simulink model "CDA"  (R2020a)
settings: Solver=VariableStepAuto  StartTime=0.0  StopTime=300  RelTol=1e-9
values from neighbouring files (symbols this model uses):
  bp = 0.05    [simulacion.m]
  kp = 3.0    (= 3)    [simulacion.m]
  kp_poc = 0.4    [simulacion.m]
  P_i_u1 = SP1    (= 180)    [simulacion.m]
  P_i_u2 = P2(1)    [simulacion.m]
  P_i_u3 = P3(1)    [simulacion.m]
  q_i_u1 = condiciones.q_i    [simulacion.m]
  q_i_u2 = condiciones.q_i    [simulacion.m]
  q_i_u3 = condiciones.q_i    [simulacion.m]
  qt_i = q_i_u1 + q_i_u2 + q_i_u3    [simulacion.m]
  SP1 = 180    [simulacion.m]
  SP2 = 180    [simulacion.m]
  SP3 = 180    [simulacion.m]
  t3 = 0.01    [simulacion.m]
  td = 0    [simulacion.m]
  tn_poc = 5    [simulacion.m]
  tx = 0.8    [simulacion.m]
  y_i_u1 = condiciones.y_i    [simulacion.m]
  y_i_u2 = condiciones.y_i    [simulacion.m]
  y_i_u3 = condiciones.y_i    [simulacion.m]
libraries: simulink x6, simulink_extras x6
settings Model: Creator=Lenovo  LastModifiedBy=Lenovo
settings SolverCC: AlgebraicLoopSolver=LineSearch

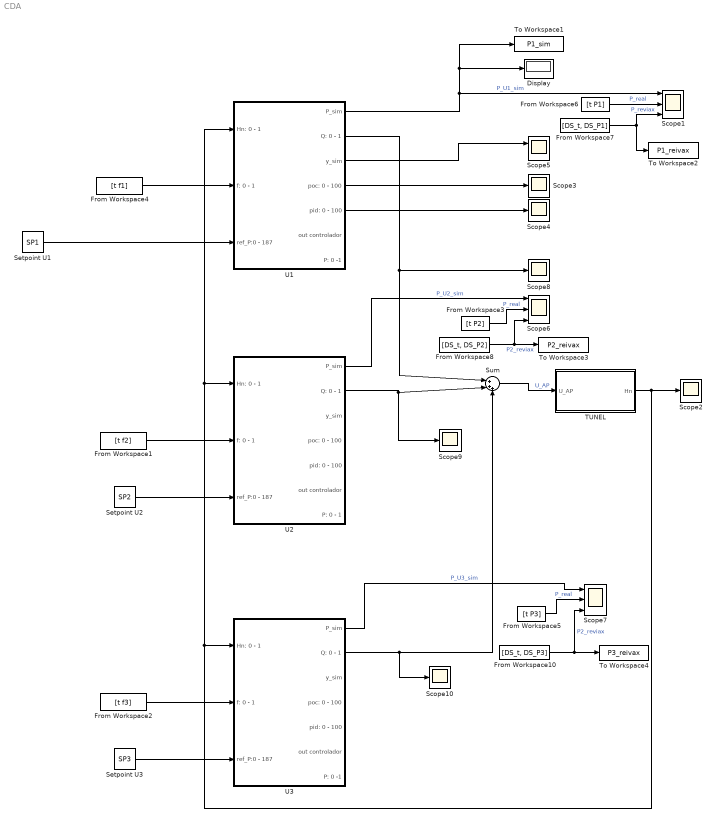
== system CDA ==
  Display : Display
  From Workspace1 : FromWorkspace  VariableName=[t f2]
  From Workspace10 : FromWorkspace  VariableName=[DS_t, DS_P3]
  From Workspace2 : FromWorkspace  VariableName=[t f3]
  From Workspace3 : FromWorkspace  VariableName=[t P2]
  From Workspace4 : FromWorkspace  VariableName=[t f1]
  From Workspace5 : FromWorkspace  VariableName=[t P3]
  From Workspace6 : FromWorkspace  VariableName=[t P1]
  From Workspace7 : FromWorkspace  VariableName=[DS_t, DS_P1]
  From Workspace8 : FromWorkspace  VariableName=[DS_t, DS_P2]
  Scope1 : Scope  NumInputPorts=3
  Scope{2..4,8..10} (6 alike) : Scope
  Scope5 : Scope  NumInputPorts=2
  Scope6 : Scope  NumInputPorts=3
  Scope7 : Scope  NumInputPorts=3
  Setpoint U1 : Constant  Value=SP1
  Setpoint U2 : Constant  Value=SP2
  Setpoint U3 : Constant  Value=SP3
  Sum : Sum  Inputs=|+++
  TUNEL : Subsystem
  To Workspace1 : ToWorkspace  VariableName=P1_sim  SaveFormat=Timeseries  SampleTime=1
  To Workspace2 : ToWorkspace  VariableName=P1_reivax  SaveFormat=Timeseries  SampleTime=1
  To Workspace3 : ToWorkspace  VariableName=P2_reivax  SaveFormat=Timeseries  SampleTime=1
  To Workspace4 : ToWorkspace  VariableName=P3_reivax  SaveFormat=Timeseries  SampleTime=1
  U1 : Subsystem
  U2 : Subsystem
  U3 : Subsystem
  wires:
  From Workspace6/1 -> Scope1/2  "P_real"
  U1/1(P_sim) -> To Workspace1/1, Display/1, Scope1/1  "P_U1_sim"
  From Workspace4/1 -> U1/2(f: 0 - 1)
  Setpoint U1/1 -> U1/3(ref_P:0 - 187)
  U1/3(y_sim) -> Scope5/1
  U1/4(poc: 0 - 100) -> Scope3/1
  U1/5(pid: 0 - 100) -> Scope4/1
  U1/2(Q: 0 - 1) -> Sum/1, Scope8/1
  U2/2(Q: 0 - 1) -> Scope9/1, Sum/2
  U3/2(Q: 0 - 1) -> Sum/3, Scope10/1
  TUNEL/1(Hn) -> Scope2/1, U1/1(Hn: 0 - 1), U2/1(Hn: 0 - 1), U3/1(Hn: 0 - 1)
  Sum/1 -> TUNEL/1(U_AP)  "U_AP"
  Setpoint U2/1 -> U2/3(ref_P:0 - 187)
  Setpoint U3/1 -> U3/3(ref_P:0 - 187)
  U2/1(P_sim) -> Scope6/1  "P_U2_sim"
  From Workspace3/1 -> Scope6/2  "P_real"
  From Workspace5/1 -> Scope7/2  "P_real"
  U3/1(P_sim) -> Scope7/1  "P_U3_sim"
  From Workspace7/1 -> Scope1/3, To Workspace2/1  "P_reviax"
  From Workspace1/1 -> U2/2(f: 0 - 1)
  From Workspace2/1 -> U3/2(f: 0 - 1)
  From Workspace8/1 -> To Workspace3/1, Scope6/3  "P2_reviax"
  From Workspace10/1 -> Scope7/3, To Workspace4/1  "P2_reviax"

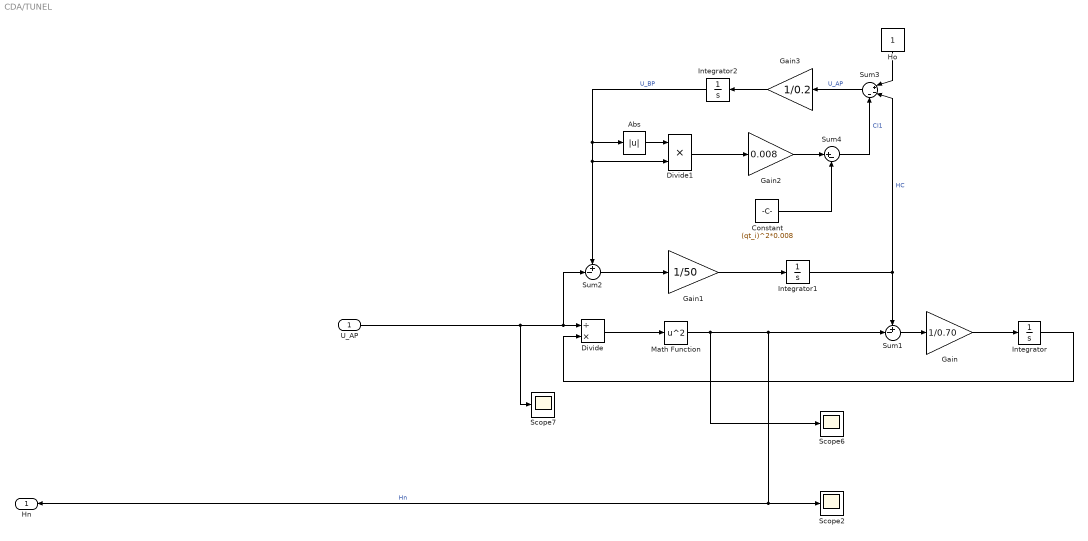
== system CDA/TUNEL ==
  U_AP : Inport
  Abs : Abs
  Constant : Constant  Value=(qt_i)^2*0.008
  Divide : Product  Inputs=/*
  Divide1 : Product  Inputs=**
  Gain : Gain  Gain=1/0.70
  Gain1 : Gain  Gain=1/50
  Gain2 : Gain  Gain=0.008
  Gain3 : Gain  Gain=1/0.2
  Ho : Constant
  Integrator : Integrator  InitialCondition=qt_i
  Integrator1 : Integrator  InitialCondition=1
  Integrator2 : Integrator  InitialCondition=qt_i
  Math Function : Math  Operator=square  SaturateOnIntegerOverflow=on
  Scope2 : Scope
  Scope6 : Scope
  Scope7 : Scope
  Sum1 : Sum  Inputs=+-|
  Sum2 : Sum  Inputs=+-|
  Sum3 : Sum  Inputs=|+--
  Sum4 : Sum  Inputs=|+-
  Hn : Outport
  wires:
  Math Function/1 -> Scope6/1, Hn/1, Scope2/1, Sum1/2  "Hn"
  Gain1/1 -> Integrator1/1
  Integrator2/1 -> Abs/1, Divide1/2, Sum2/1  "U_BP"
  Ho/1 -> Sum3/1
  Integrator/1 -> Divide/2
  Gain/1 -> Integrator/1
  Divide/1 -> Math Function/1
  Sum4/1 -> Sum3/3  "CI1"
  U_AP/1 -> Scope7/1, Sum2/2, Divide/1
  Gain2/1 -> Sum4/1
  Integrator1/1 -> Sum3/2, Sum1/1  "HC"
  Constant/1 -> Sum4/2
  Sum1/1 -> Gain/1
  Gain3/1 -> Integrator2/1
  Sum2/1 -> Gain1/1
  Divide1/1 -> Gain2/1
  Sum3/1 -> Gain3/1  "U_AP"
  Abs/1 -> Divide1/1

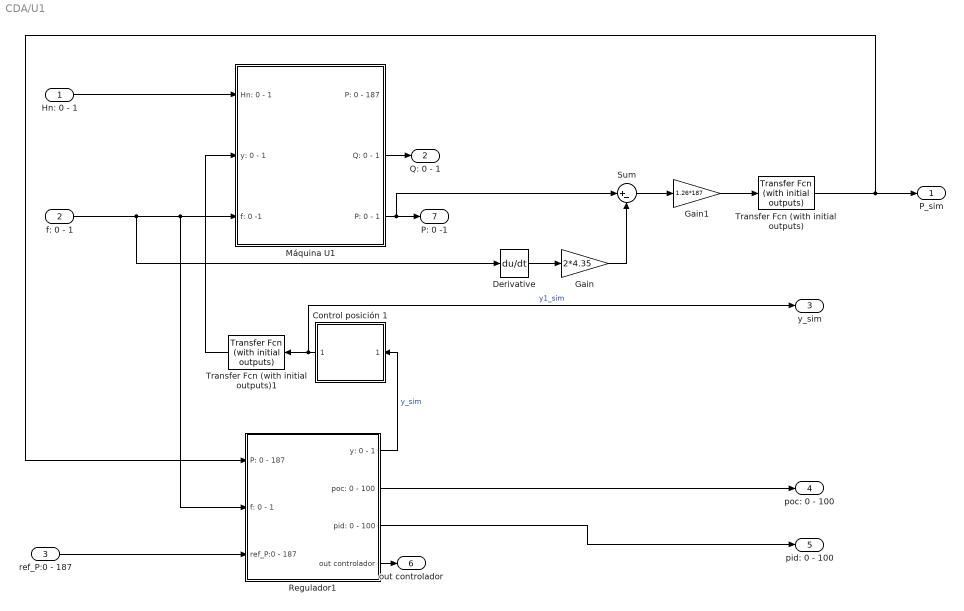
== system CDA/U1 ==
  Hn: 0 - 1 : Inport
  f: 0 - 1 : Inport  Port=2
  ref_P:0 - 187 : Inport  Port=3
  Control posición 1 : Subsystem
  Derivative : Derivative
  Gain : Gain  Gain=2*4.35
  Gain1 : Gain  Gain=1.26*187
  Máquina U1 : Subsystem
  Regulador1 : Subsystem
  Sum : Sum  Inputs=|+-
  Transfer Fcn (with initial outputs) : simulink_extras/Additional Linear/Transfer Fcn (with initial outputs)  N=[1]  D="[0.2  1]"  Y0=P_i_u1  U0=P_i_u1/(1.26*187)
  Transfer Fcn (with initial outputs)1 : simulink_extras/Additional Linear/Transfer Fcn (with initial outputs)  N=[1]  D=[1e-6 1]  Y0=y_i_u1  U0=y_i_u1
  P_sim : Outport
  Q: 0 - 1 : Outport  Port=2
  y_sim : Outport  Port=3
  poc: 0 - 100 : Outport  Port=4
  pid: 0 - 100 : Outport  Port=5
  out controlador : Outport  Port=6
  P: 0 -1 : Outport  Port=7
  wires:
  Control posición 1/1(yr: 0 - 1) -> Transfer Fcn (with initial outputs)1/1, y_sim/1  "y1_sim"
  Regulador1/1(y: 0 - 1) -> Control posición 1/1(yf: 0 - 1)  "y_sim"
  Máquina U1/2(Q: 0 - 1) -> Q: 0 - 1/1
  ref_P:0 - 187/1 -> Regulador1/3(ref_P:0 - 187)
  Hn: 0 - 1/1 -> Máquina U1/1(Hn: 0 - 1)
  f: 0 - 1/1 -> Derivative/1, Máquina U1/3(f: 0 -1), Regulador1/2(f: 0 - 1)
  Transfer Fcn (with initial outputs)1/1 -> Máquina U1/2(y: 0 - 1)
  Regulador1/3(pid: 0 - 100) -> pid: 0 - 100/1
  Regulador1/2(poc: 0 - 100) -> poc: 0 - 100/1
  Regulador1/4(out controlador) -> out controlador/1
  Máquina U1/3(P: 0 - 1) -> Sum/1, P: 0 -1/1
  Derivative/1 -> Gain/1
  Gain/1 -> Sum/2
  Sum/1 -> Gain1/1
  Gain1/1 -> Transfer Fcn (with initial outputs)/1
  Transfer Fcn (with initial outputs)/1 -> Regulador1/1(P: 0 - 187), P_sim/1

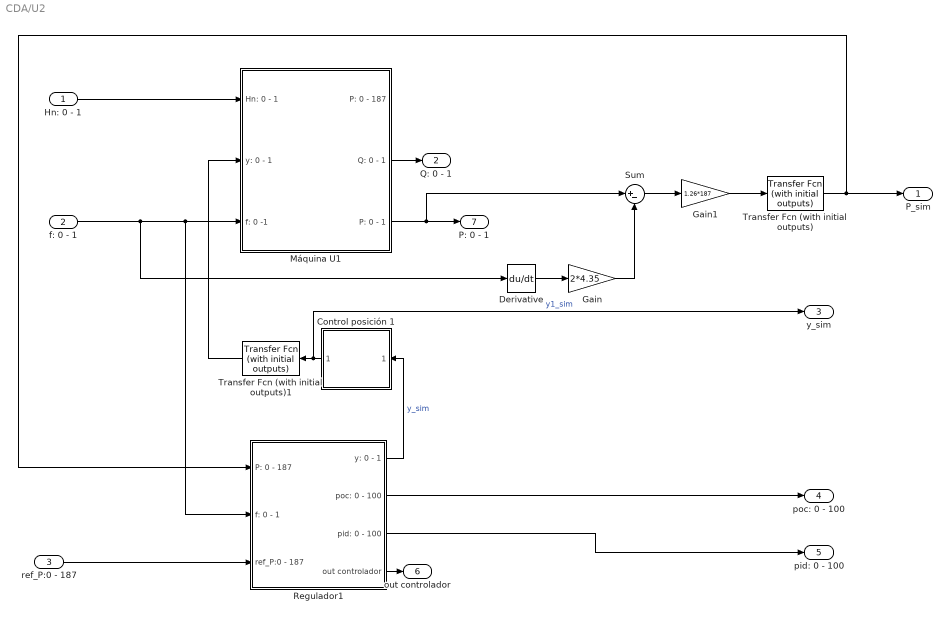
== system CDA/U2 ==
  Hn: 0 - 1 : Inport
  f: 0 - 1 : Inport  Port=2
  ref_P:0 - 187 : Inport  Port=3
  Control posición 1 : Subsystem
  Derivative : Derivative
  Gain : Gain  Gain=2*4.35
  Gain1 : Gain  Gain=1.26*187
  Máquina U1 : Subsystem
  Regulador1 : Subsystem
  Sum : Sum  Inputs=|+-
  Transfer Fcn (with initial outputs) : simulink_extras/Additional Linear/Transfer Fcn (with initial outputs)  N=[1]  D="[0.2  1]"  Y0=P_i_u2  U0=P_i_u2/(1.26*187)
  Transfer Fcn (with initial outputs)1 : simulink_extras/Additional Linear/Transfer Fcn (with initial outputs)  N=[1]  D=[1e-6 1]  Y0=y_i_u2  U0=y_i_u2
  P_sim : Outport
  Q: 0 - 1 : Outport  Port=2
  y_sim : Outport  Port=3
  poc: 0 - 100 : Outport  Port=4
  pid: 0 - 100 : Outport  Port=5
  out controlador : Outport  Port=6
  P: 0 - 1 : Outport  Port=7
  wires:
  Control posición 1/1(yr: 0 - 1) -> Transfer Fcn (with initial outputs)1/1, y_sim/1  "y1_sim"
  Regulador1/1(y: 0 - 1) -> Control posición 1/1(yf: 0 - 1)  "y_sim"
  Máquina U1/2(Q: 0 - 1) -> Q: 0 - 1/1
  ref_P:0 - 187/1 -> Regulador1/3(ref_P:0 - 187)
  Hn: 0 - 1/1 -> Máquina U1/1(Hn: 0 - 1)
  Transfer Fcn (with initial outputs)1/1 -> Máquina U1/2(y: 0 - 1)
  Regulador1/3(pid: 0 - 100) -> pid: 0 - 100/1
  Regulador1/2(poc: 0 - 100) -> poc: 0 - 100/1
  Regulador1/4(out controlador) -> out controlador/1
  Máquina U1/3(P: 0 - 1) -> Sum/1, P: 0 - 1/1
  Sum/1 -> Gain1/1
  Gain/1 -> Sum/2
  Derivative/1 -> Gain/1
  f: 0 - 1/1 -> Derivative/1, Máquina U1/3(f: 0 -1), Regulador1/2(f: 0 - 1)
  Gain1/1 -> Transfer Fcn (with initial outputs)/1
  Transfer Fcn (with initial outputs)/1 -> P_sim/1, Regulador1/1(P: 0 - 187)

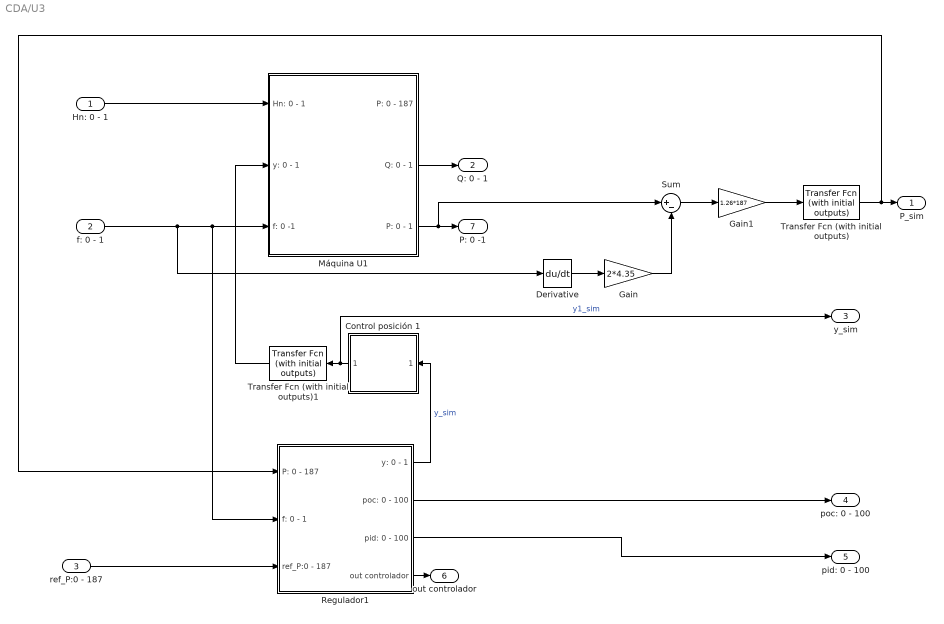
== system CDA/U3 ==
  Hn: 0 - 1 : Inport
  f: 0 - 1 : Inport  Port=2
  ref_P:0 - 187 : Inport  Port=3
  Control posición 1 : Subsystem
  Derivative : Derivative
  Gain : Gain  Gain=2*4.35
  Gain1 : Gain  Gain=1.26*187
  Máquina U1 : Subsystem
  Regulador1 : Subsystem
  Sum : Sum  Inputs=|+-
  Transfer Fcn (with initial outputs) : simulink_extras/Additional Linear/Transfer Fcn (with initial outputs)  N=[1]  D="[0.2  1]"  Y0=P_i_u3  U0=P_i_u3/(1.26*187)
  Transfer Fcn (with initial outputs)1 : simulink_extras/Additional Linear/Transfer Fcn (with initial outputs)  N=[1]  D=[1e-6 1]  Y0=y_i_u3  U0=y_i_u3
  P_sim : Outport
  Q: 0 - 1 : Outport  Port=2
  y_sim : Outport  Port=3
  poc: 0 - 100 : Outport  Port=4
  pid: 0 - 100 : Outport  Port=5
  out controlador : Outport  Port=6
  P: 0 -1 : Outport  Port=7
  wires:
  Control posición 1/1(yr: 0 - 1) -> Transfer Fcn (with initial outputs)1/1, y_sim/1  "y1_sim"
  Regulador1/1(y: 0 - 1) -> Control posición 1/1(yf: 0 - 1)  "y_sim"
  Máquina U1/2(Q: 0 - 1) -> Q: 0 - 1/1
  ref_P:0 - 187/1 -> Regulador1/3(ref_P:0 - 187)
  Hn: 0 - 1/1 -> Máquina U1/1(Hn: 0 - 1)
  Transfer Fcn (with initial outputs)1/1 -> Máquina U1/2(y: 0 - 1)
  Regulador1/3(pid: 0 - 100) -> pid: 0 - 100/1
  Regulador1/2(poc: 0 - 100) -> poc: 0 - 100/1
  Regulador1/4(out controlador) -> out controlador/1
  Máquina U1/3(P: 0 - 1) -> Sum/1, P: 0 -1/1
  Sum/1 -> Gain1/1
  Gain/1 -> Sum/2
  Derivative/1 -> Gain/1
  f: 0 - 1/1 -> Derivative/1, Máquina U1/3(f: 0 -1), Regulador1/2(f: 0 - 1)
  Gain1/1 -> Transfer Fcn (with initial outputs)/1
  Transfer Fcn (with initial outputs)/1 -> Regulador1/1(P: 0 - 187), P_sim/1

== system CDA/U1/Control posición 1 ==
  yf: 0 - 1 : Inport
  Gain : Gain  Gain=15
  Gain1 : Gain  Gain=0.3
  Gain2 : Gain  Gain=1/100
  Gain3 : Gain  Gain=100
  Gain4 : Gain  Gain=100
  Integrator : Integrator  InitialCondition=y_i_u1  LimitOutput=on  UpperSaturationLimit=1  LowerSaturationLimit=-1
  Saturation : Saturate  UpperLimit=100  LowerLimit=-100
  Saturation1 : Saturate  UpperLimit=0.1  LowerLimit=-0.1
  Sum : Sum  Inputs=|+-
  Transfer Fcn : TransferFcn  Denominator=[0.020 1]
  yr: 0 - 1 : Outport
  wires:
  Gain4/1 -> Sum/1
  yf: 0 - 1/1 -> Gain4/1
  Saturation1/1 -> Integrator/1
  Gain1/1 -> Saturation1/1
  Sum/1 -> Gain/1
  Transfer Fcn/1 -> Gain1/1
  Gain/1 -> Saturation/1
  Gain3/1 -> Sum/2
  Saturation/1 -> Gain2/1
  Gain2/1 -> Transfer Fcn/1
  Integrator/1 -> Gain3/1, yr: 0 - 1/1

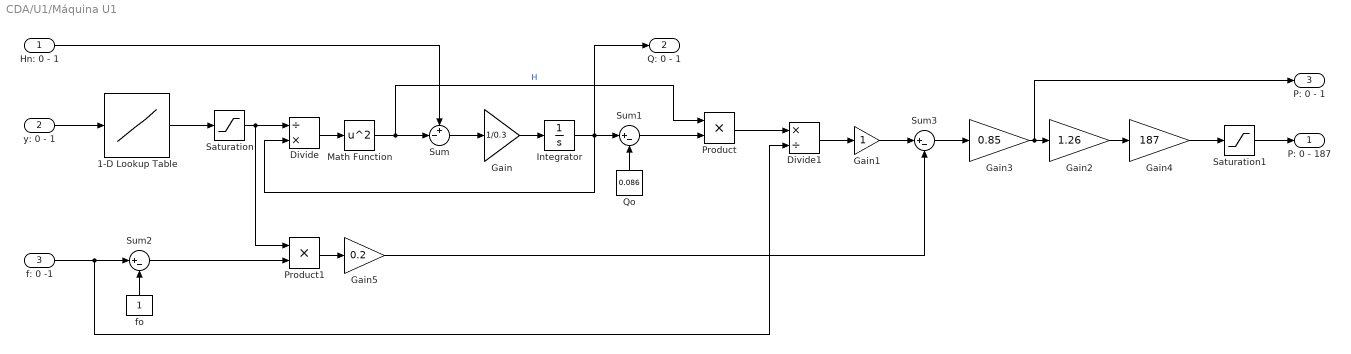
== system CDA/U1/Máquina U1 ==
  Hn: 0 - 1 : Inport
  y: 0 - 1 : Inport  Port=2
  f: 0 -1 : Inport  Port=3
  1-D Lookup Table : Lookup_n-D  NumberOfTableDimensions=1  BreakpointsForDimension1=[0,0.072,0.336,0.35,0.4,0.45,0.5,0.55,0.6,0.65,0.7,0.75,0.8,0.85,0.9,0.95,1]  Table=[0,0.086,0.387,0.4035,0.4592,0.5194,0.5826,0.6475,0.7127,0.777,0.8389,0.8971,0.9502,0.9969,1.0358,1.0656,1.0849]  InternalRulePriority=Speed  RndMeth=Simplest  InputSameDT=on
  Divide : Product  Inputs=/*
  Divide1 : Product  Inputs=*/
  Gain : Gain  Gain=1/0.3
  Gain1 : Gain
  Gain2 : Gain  Gain=1.26
  Gain3 : Gain  Gain=0.85
  Gain4 : Gain  Gain=187
  Gain5 : Gain  Gain=0.2
  Integrator : Integrator  InitialCondition=q_i_u1
  Math Function : Math  Operator=square  SaturateOnIntegerOverflow=on
  Product : Product
  Product1 : Product
  Qo : Constant  Value=0.086
  Saturation : Saturate  UpperLimit=1.1  LowerLimit=0.0001
  Saturation1 : Saturate  UpperLimit=200  LowerLimit=0
  Sum : Sum  Inputs=+-|
  Sum1 : Sum  Inputs=|+-
  Sum2 : Sum  Inputs=|+-
  Sum3 : Sum  Inputs=|+-
  fo : Constant
  P: 0 - 187 : Outport
  Q: 0 - 1 : Outport  Port=2
  P: 0 - 1 : Outport  Port=3
  wires:
  Math Function/1 -> Sum/2, Product/1  "H"
  Integrator/1 -> Q: 0 - 1/1, Sum1/1, Divide/2
  Qo/1 -> Sum1/2
  Gain2/1 -> Gain4/1
  y: 0 - 1/1 -> 1-D Lookup Table/1
  Saturation/1 -> Divide/1, Product1/1
  1-D Lookup Table/1 -> Saturation/1
  f: 0 -1/1 -> Divide1/2, Sum2/1
  Gain1/1 -> Sum3/1
  Sum1/1 -> Product/2
  Product1/1 -> Gain5/1
  Divide1/1 -> Gain1/1
  Sum2/1 -> Product1/2
  Divide/1 -> Math Function/1
  Product/1 -> Divide1/1
  Hn: 0 - 1/1 -> Sum/1
  Gain5/1 -> Sum3/2
  Sum3/1 -> Gain3/1
  Sum/1 -> Gain/1
  Gain/1 -> Integrator/1
  Gain3/1 -> P: 0 - 1/1, Gain2/1
  fo/1 -> Sum2/2
  Gain4/1 -> Saturation1/1
  Saturation1/1 -> P: 0 - 187/1

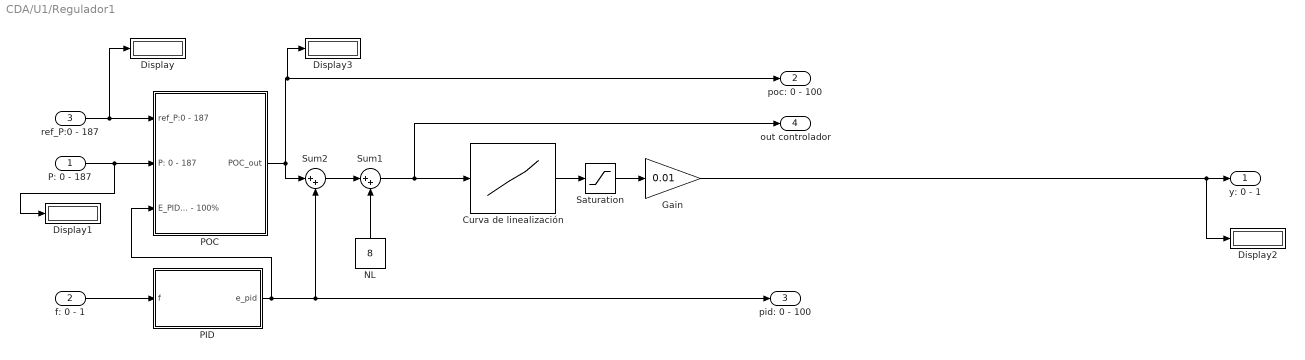
== system CDA/U1/Regulador1 ==
  P: 0 - 187 : Inport
  f: 0 - 1 : Inport  Port=2
  ref_P:0 - 187 : Inport  Port=3
  Curva de linealización : Lookup_n-D  NumberOfTableDimensions=1  BreakpointsForDimension1=[-1,0,8,8.001,18,38,48,58,68,78,88,98,107,151]  Table=[-1,0,8,8.001,17.4,33.1,40,46.3,51.8,59.0,67,78,89,115]  InternalRulePriority=Speed  RndMeth=Simplest  InputSameDT=on
  Display{,1..3} (4 alike) : Display
  Gain : Gain  Gain=0.01
  NL : Constant  Value=8
  PID : Subsystem
  POC : Subsystem
  Saturation : Saturate  UpperLimit=115  LowerLimit=7.9  ZeroCross=off
  Sum1 : Sum  Inputs=|++
  Sum2 : Sum  Inputs=|++
  y: 0 - 1 : Outport
  poc: 0 - 100 : Outport  Port=2
  pid: 0 - 100 : Outport  Port=3
  out controlador : Outport  Port=4
  wires:
  PID/1(e_pid) -> POC/3(E_PID: 0 - 100%), Sum2/2, pid: 0 - 100/1
  POC/1(POC_out) -> Display3/1, poc: 0 - 100/1, Sum2/1
  f: 0 - 1/1 -> PID/1(f)
  NL/1 -> Sum1/2
  Sum2/1 -> Sum1/1
  ref_P:0 - 187/1 -> Display/1, POC/1(ref_P:0 - 187)
  P: 0 - 187/1 -> Display1/1, POC/2(P: 0 - 187)
  Saturation/1 -> Gain/1
  Curva de linealización/1 -> Saturation/1
  Gain/1 -> Display2/1, y: 0 - 1/1
  Sum1/1 -> out controlador/1, Curva de linealización/1

== system CDA/U2/Control posición 1 ==
  yf: 0 - 1 : Inport
  Gain : Gain  Gain=15
  Gain1 : Gain  Gain=0.3
  Gain2 : Gain  Gain=1/100
  Gain3 : Gain  Gain=100
  Gain4 : Gain  Gain=100
  Integrator : Integrator  InitialCondition=y_i_u2  LimitOutput=on  UpperSaturationLimit=1  LowerSaturationLimit=-1
  Saturation : Saturate  UpperLimit=100  LowerLimit=-100
  Saturation1 : Saturate  UpperLimit=0.1  LowerLimit=-0.1
  Sum : Sum  Inputs=|+-
  Transfer Fcn : TransferFcn  Denominator=[0.020 1]
  yr: 0 - 1 : Outport
  wires:
  Gain4/1 -> Sum/1
  yf: 0 - 1/1 -> Gain4/1
  Saturation1/1 -> Integrator/1
  Gain1/1 -> Saturation1/1
  Sum/1 -> Gain/1
  Transfer Fcn/1 -> Gain1/1
  Gain/1 -> Saturation/1
  Gain3/1 -> Sum/2
  Saturation/1 -> Gain2/1
  Gain2/1 -> Transfer Fcn/1
  Integrator/1 -> Gain3/1, yr: 0 - 1/1

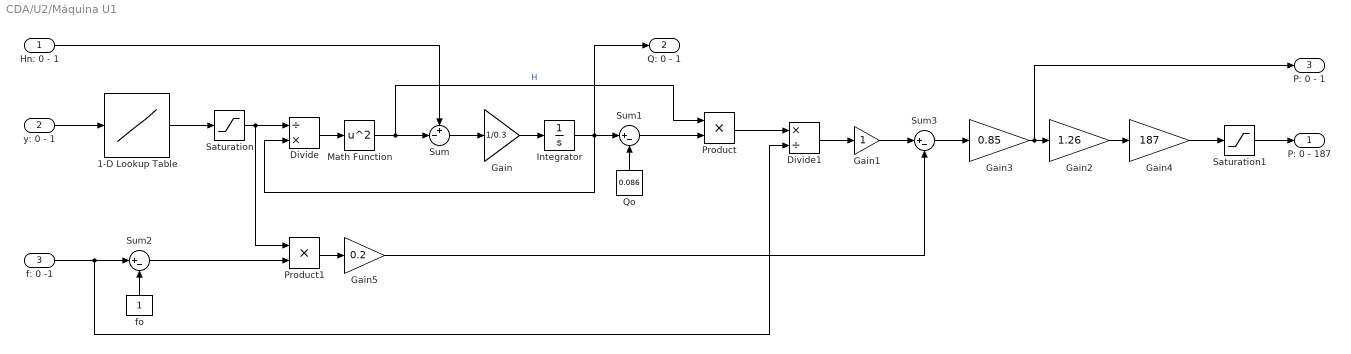
== system CDA/U2/Máquina U1 ==
  Hn: 0 - 1 : Inport
  y: 0 - 1 : Inport  Port=2
  f: 0 -1 : Inport  Port=3
  1-D Lookup Table : Lookup_n-D  NumberOfTableDimensions=1  BreakpointsForDimension1=[0,0.072,0.336,0.35,0.4,0.45,0.5,0.55,0.6,0.65,0.7,0.75,0.8,0.85,0.9,0.95,1]  Table=[0,0.086,0.387,0.4035,0.4592,0.5194,0.5826,0.6475,0.7127,0.777,0.8389,0.8971,0.9502,0.9969,1.0358,1.0656,1.0849]  InternalRulePriority=Speed  RndMeth=Simplest  InputSameDT=on
  Divide : Product  Inputs=/*
  Divide1 : Product  Inputs=*/
  Gain : Gain  Gain=1/0.3
  Gain1 : Gain
  Gain2 : Gain  Gain=1.26
  Gain3 : Gain  Gain=0.85
  Gain4 : Gain  Gain=187
  Gain5 : Gain  Gain=0.2
  Integrator : Integrator  InitialCondition=q_i_u2
  Math Function : Math  Operator=square  SaturateOnIntegerOverflow=on
  Product : Product
  Product1 : Product
  Qo : Constant  Value=0.086
  Saturation : Saturate  UpperLimit=1.1  LowerLimit=0.0001
  Saturation1 : Saturate  UpperLimit=200  LowerLimit=0
  Sum : Sum  Inputs=+-|
  Sum1 : Sum  Inputs=|+-
  Sum2 : Sum  Inputs=|+-
  Sum3 : Sum  Inputs=|+-
  fo : Constant
  P: 0 - 187 : Outport
  Q: 0 - 1 : Outport  Port=2
  P: 0 - 1 : Outport  Port=3
  wires:
  Math Function/1 -> Sum/2, Product/1  "H"
  Integrator/1 -> Q: 0 - 1/1, Sum1/1, Divide/2
  Qo/1 -> Sum1/2
  Gain2/1 -> Gain4/1
  y: 0 - 1/1 -> 1-D Lookup Table/1
  Saturation/1 -> Divide/1, Product1/1
  1-D Lookup Table/1 -> Saturation/1
  f: 0 -1/1 -> Divide1/2, Sum2/1
  Gain1/1 -> Sum3/1
  Sum1/1 -> Product/2
  Product1/1 -> Gain5/1
  Divide1/1 -> Gain1/1
  Sum2/1 -> Product1/2
  Divide/1 -> Math Function/1
  Product/1 -> Divide1/1
  Hn: 0 - 1/1 -> Sum/1
  Gain5/1 -> Sum3/2
  Sum3/1 -> Gain3/1
  Sum/1 -> Gain/1
  Gain/1 -> Integrator/1
  Gain3/1 -> P: 0 - 1/1, Gain2/1
  fo/1 -> Sum2/2
  Gain4/1 -> Saturation1/1
  Saturation1/1 -> P: 0 - 187/1

== system CDA/U2/Regulador1 ==
  P: 0 - 187 : Inport
  f: 0 - 1 : Inport  Port=2
  ref_P:0 - 187 : Inport  Port=3
  Curva de linealización : Lookup_n-D  NumberOfTableDimensions=1  BreakpointsForDimension1=[-1,0,8,8.001,18,38,48,58,68,78,88,98,107,151]  Table=[-1,0,8,8.001,17.4,33.1,40,46.3,51.8,59.0,67,78,89,115]  InternalRulePriority=Speed  RndMeth=Simplest  InputSameDT=on
  Display{,1..3} (4 alike) : Display
  Gain : Gain  Gain=0.01
  NL : Constant  Value=8
  PID : Subsystem
  POC : Subsystem
  Saturation : Saturate  UpperLimit=115  LowerLimit=7.9  ZeroCross=off
  Sum1 : Sum  Inputs=|++
  Sum2 : Sum  Inputs=|++
  y: 0 - 1 : Outport
  poc: 0 - 100 : Outport  Port=2
  pid: 0 - 100 : Outport  Port=3
  out controlador : Outport  Port=4
  wires:
  PID/1(e_pid) -> POC/3(E_PID: 0 - 100%), Sum2/2, pid: 0 - 100/1
  POC/1(POC_out) -> Display3/1, poc: 0 - 100/1, Sum2/1
  f: 0 - 1/1 -> PID/1(f)
  NL/1 -> Sum1/2
  Sum2/1 -> Sum1/1
  ref_P:0 - 187/1 -> Display/1, POC/1(ref_P:0 - 187)
  P: 0 - 187/1 -> Display1/1, POC/2(P: 0 - 187)
  Saturation/1 -> Gain/1
  Curva de linealización/1 -> Saturation/1
  Gain/1 -> Display2/1, y: 0 - 1/1
  Sum1/1 -> out controlador/1, Curva de linealización/1

== system CDA/U3/Control posición 1 ==
  yf: 0 - 1 : Inport
  Gain : Gain  Gain=15
  Gain1 : Gain  Gain=0.3
  Gain2 : Gain  Gain=1/100
  Gain3 : Gain  Gain=100
  Gain4 : Gain  Gain=100
  Integrator : Integrator  InitialCondition=y_i_u3  LimitOutput=on  UpperSaturationLimit=1  LowerSaturationLimit=-1
  Saturation : Saturate  UpperLimit=100  LowerLimit=-100
  Saturation1 : Saturate  UpperLimit=0.1  LowerLimit=-0.1
  Sum : Sum  Inputs=|+-
  Transfer Fcn : TransferFcn  Denominator=[0.020 1]
  yr: 0 - 1 : Outport
  wires:
  Gain4/1 -> Sum/1
  yf: 0 - 1/1 -> Gain4/1
  Saturation1/1 -> Integrator/1
  Gain1/1 -> Saturation1/1
  Sum/1 -> Gain/1
  Transfer Fcn/1 -> Gain1/1
  Gain/1 -> Saturation/1
  Gain3/1 -> Sum/2
  Saturation/1 -> Gain2/1
  Gain2/1 -> Transfer Fcn/1
  Integrator/1 -> Gain3/1, yr: 0 - 1/1

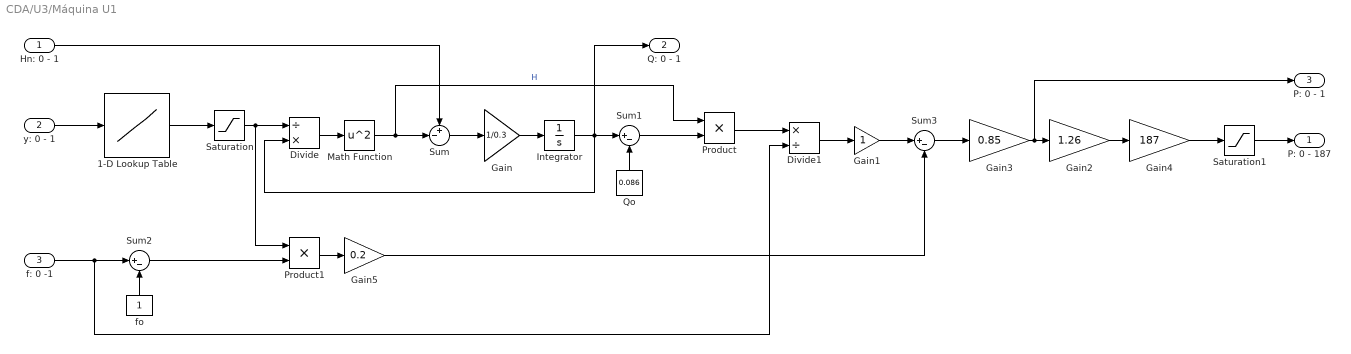
== system CDA/U3/Máquina U1 ==
  Hn: 0 - 1 : Inport
  y: 0 - 1 : Inport  Port=2
  f: 0 -1 : Inport  Port=3
  1-D Lookup Table : Lookup_n-D  NumberOfTableDimensions=1  BreakpointsForDimension1=[0,0.072,0.336,0.35,0.4,0.45,0.5,0.55,0.6,0.65,0.7,0.75,0.8,0.85,0.9,0.95,1]  Table=[0,0.086,0.387,0.4035,0.4592,0.5194,0.5826,0.6475,0.7127,0.777,0.8389,0.8971,0.9502,0.9969,1.0358,1.0656,1.0849]  InternalRulePriority=Speed  RndMeth=Simplest  InputSameDT=on
  Divide : Product  Inputs=/*
  Divide1 : Product  Inputs=*/
  Gain : Gain  Gain=1/0.3
  Gain1 : Gain
  Gain2 : Gain  Gain=1.26
  Gain3 : Gain  Gain=0.85
  Gain4 : Gain  Gain=187
  Gain5 : Gain  Gain=0.2
  Integrator : Integrator  InitialCondition=q_i_u3
  Math Function : Math  Operator=square  SaturateOnIntegerOverflow=on
  Product : Product
  Product1 : Product
  Qo : Constant  Value=0.086
  Saturation : Saturate  UpperLimit=1.1  LowerLimit=0.0001
  Saturation1 : Saturate  UpperLimit=200  LowerLimit=0
  Sum : Sum  Inputs=+-|
  Sum1 : Sum  Inputs=|+-
  Sum2 : Sum  Inputs=|+-
  Sum3 : Sum  Inputs=|+-
  fo : Constant
  P: 0 - 187 : Outport
  Q: 0 - 1 : Outport  Port=2
  P: 0 - 1 : Outport  Port=3
  wires:
  Math Function/1 -> Sum/2, Product/1  "H"
  Integrator/1 -> Q: 0 - 1/1, Sum1/1, Divide/2
  Qo/1 -> Sum1/2
  Gain2/1 -> Gain4/1
  y: 0 - 1/1 -> 1-D Lookup Table/1
  Saturation/1 -> Divide/1, Product1/1
  1-D Lookup Table/1 -> Saturation/1
  f: 0 -1/1 -> Divide1/2, Sum2/1
  Gain1/1 -> Sum3/1
  Sum1/1 -> Product/2
  Product1/1 -> Gain5/1
  Divide1/1 -> Gain1/1
  Sum2/1 -> Product1/2
  Divide/1 -> Math Function/1
  Product/1 -> Divide1/1
  Hn: 0 - 1/1 -> Sum/1
  Gain5/1 -> Sum3/2
  Sum3/1 -> Gain3/1
  Sum/1 -> Gain/1
  Gain/1 -> Integrator/1
  Gain3/1 -> P: 0 - 1/1, Gain2/1
  fo/1 -> Sum2/2
  Gain4/1 -> Saturation1/1
  Saturation1/1 -> P: 0 - 187/1

== system CDA/U3/Regulador1 ==
  P: 0 - 187 : Inport
  f: 0 - 1 : Inport  Port=2
  ref_P:0 - 187 : Inport  Port=3
  Curva de linealización : Lookup_n-D  NumberOfTableDimensions=1  BreakpointsForDimension1=[-1,0,8,8.001,18,38,48,58,68,78,88,98,107,151]  Table=[-1,0,8,8.001,17.4,33.1,40,46.3,51.8,59.0,67,78,89,115]  InternalRulePriority=Speed  RndMeth=Simplest  InputSameDT=on
  Display{,1..3} (4 alike) : Display
  Gain : Gain  Gain=0.01
  NL : Constant  Value=8
  PID : Subsystem
  POC : Subsystem
  Saturation : Saturate  UpperLimit=115  LowerLimit=7.9  ZeroCross=off
  Sum1 : Sum  Inputs=|++
  Sum2 : Sum  Inputs=|++
  y: 0 - 1 : Outport
  poc: 0 - 100 : Outport  Port=2
  pid: 0 - 100 : Outport  Port=3
  out controlador : Outport  Port=4
  wires:
  PID/1(e_pid) -> POC/3(E_PID: 0 - 100%), Sum2/2, pid: 0 - 100/1
  POC/1(POC_out) -> Display3/1, poc: 0 - 100/1, Sum2/1
  f: 0 - 1/1 -> PID/1(f)
  NL/1 -> Sum1/2
  Sum2/1 -> Sum1/1
  ref_P:0 - 187/1 -> Display/1, POC/1(ref_P:0 - 187)
  P: 0 - 187/1 -> Display1/1, POC/2(P: 0 - 187)
  Saturation/1 -> Gain/1
  Curva de linealización/1 -> Saturation/1
  Gain/1 -> Display2/1, y: 0 - 1/1
  Sum1/1 -> out controlador/1, Curva de linealización/1

== system CDA/U1/Regulador1/PID ==
  f : Inport
  Dead Zone : DeadZone  LowerValue=100-0.01  UpperValue=100+0.01  SaturateOnIntegerOverflow=on
  Derivative : Derivative
  Gain : Gain  Gain=1/tx
  Gain1 : Gain  Gain=kp
  Gain2 : Gain  Gain=td
  Gain3 : Gain  Gain=bp
  Gain4 : Gain  Gain=-1
  Gain5 : Gain  Gain=100
  IC1 : InitialCondition  Value=100
  Integrator : Integrator
  Saturation : Saturate  UpperLimit=2.5  LowerLimit=-2.5
  Sum1 : Sum  Inputs=++|
  Sum2 : Sum  Inputs=++|
  Sum3 : Sum  Inputs=|+-
  Transfer Fcn1 : TransferFcn  Denominator=[t3 1]
  e_pid : Outport
  wires:
  Saturation/1 -> e_pid/1
  Transfer Fcn1/1 -> Integrator/1, Gain2/1
  Gain2/1 -> Sum2/1
  Sum1/1 -> Transfer Fcn1/1
  Dead Zone/1 -> Gain4/1
  Integrator/1 -> Sum2/2, Gain3/1
  Gain3/1 -> Sum3/2
  f/1 -> Gain5/1
  Derivative/1 -> Gain1/1
  IC1/1 -> Dead Zone/1
  Gain4/1 -> Sum3/1, Derivative/1
  Gain/1 -> Sum1/2
  Gain1/1 -> Sum1/1
  Sum2/1 -> Saturation/1
  Sum3/1 -> Gain/1
  Gain5/1 -> IC1/1

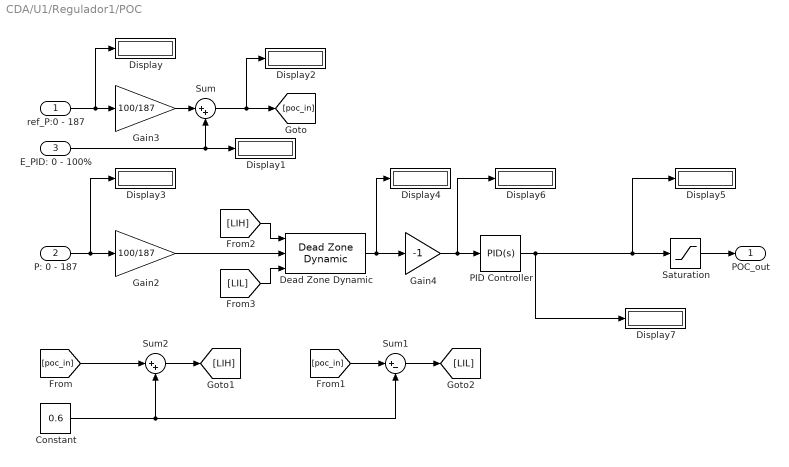
== system CDA/U1/Regulador1/POC ==
  ref_P:0 - 187 : Inport
  P: 0 - 187 : Inport  Port=2
  E_PID: 0 - 100% : Inport  Port=3
  Constant : Constant  Value=0.6
  Dead Zone Dynamic : simulink/Discontinuities/Dead Zone Dynamic
      settings: SourceProductBaseCode=SL
  Display{,1..7} (8 alike) : Display
  Gain2 : Gain  Gain=100/187
  Gain3 : Gain  Gain=100/187
  Gain4 : Gain  Gain=-1
  PID Controller : simulink/Continuous/PID Controller  Controller=PID  Form=Parallel  TimeDomain=Continuous-time  UseExternalTs=off  SampleTime=-1  IntegratorMethod=Forward Euler  FilterMethod=Forward Euler  ControllerParametersSource=internal  P=kp_poc  I=kp_poc/tn_poc  D=0  UseFilter=on  N=100  TunerSelectOption=Transfer Function Based (PID Tuner App)  InitialConditionSource=internal  InitialConditionForIntegrator=poc_i_u1  InitialConditionForFilter=0  DifferentiatorICPrevScaledInput=0  ExternalReset=none  TrackingMode=off  Kt=1  LimitOutput=off  UpperSaturationLimit=inf  LowerSaturationLimit=-inf  LinearizeAsGain=on  AntiWindupMode=none  Kb=1  POutMin=[]  POutMax=[]  IOutMin=[]  IOutMax=[]  DOutMin=[]  DOutMax=[]  NOutMin=[]  NOutMax=[]  SumOutMin=[]  SumOutMax=[]  SaturationOutMin=[]  SaturationOutMax=[]  PParamMin=[]  PParamMax=[]  IParamMin=[]  IParamMax=[]  DParamMin=[]  DParamMax=[]  NParamMin=[]  NParamMax=[]  KbParamMin=[]  KbParamMax=[]  KtParamMin=[]  KtParamMax=[]  KbOutMin=[]  KbOutMax=[]  KtOutMin=[]  KtOutMax=[]  IntegratorOutMin=[]  IntegratorOutMax=[]  FilterOutMin=[]  FilterOutMax=[]  SumI1OutMin=[]  SumI1OutMax=[]  SumI2OutMin=[]  SumI2OutMax=[]  SumI3OutMin=[]  SumI3OutMax=[]  SumI4OutMin=[]  SumI4OutMax=[]  SumDOutMin=[]  SumDOutMax=[]  DifferentiatorOutMin=[]  DifferentiatorOutMax=[]  FilterDiffOutCoefMin=[]  FilterDiffOutCoefMax=[]  ReciprocalOutMin=[]  ReciprocalOutMax=[]  SumDenOutMin=[]  SumDenOutMax=[]  SumNumOutMin=[]  SumNumOutMax=[]  DivideOutMin=[]  DivideOutMax=[]  UdiffTsProdOutMin=[]  UdiffTsProdOutMax=[]  NTsProdOutMin=[]  NTsProdOutMax=[]  UintegralTsProdOutMin=[]  UintegralTsProdOutMax=[]  UngainTsProdOutMin=[]  UngainTsProdOutMax=[]  IntegratorContinuousStateAttributes=''  IntegratorStateMustResolveToSignalObject=off  IntegratorRTWStateStorageClass=Auto  FilterContinuousStateAttributes=''  FilterStateMustResolveToSignalObject=off  FilterRTWStateStorageClass=Auto  ParallelPVariant=InternalParameters  IdealPVariant=Disabled  IVariant=InternalParameters  DVariant=InternalParameters  IntegratorVariant=Continuous  SatVariant=Disabled  AWVariant=Passthrough  PCopyVariant=Disabled  TRVariant=Disabled  FdbkBlocksVariant=Forward  IdealPFdbkVariant=Disabled  SatFdbkVariant=Disabled  DerivativeFilterVariant=ContFilter  NVariant=InternalParameters  NCopyVariant=Disabled  FilterICVariant=InternalICsFilter  IntegratorICVariant=InternalICs  ExternalResetVariant=Disabled  TRSumVariant=Passthrough  SumFdbkVariant=Disabled  SumVariant=Sum_PID  TsampFilterVariant=InternalTs  TsampNgainVariant=Passthrough  TsampIntegralVariant=Passthrough
  Saturation : Saturate  UpperLimit=120  LowerLimit=-120  ZeroCross=off
  Sum : Sum  Inputs=|++
  Sum1 : Sum  Inputs=|+-
  Sum2 : Sum  Inputs=|++
  POC_out : Outport
  wires:
  Sum2/1 -> [LIH]
  [LIL] -> Dead Zone Dynamic/3
  Gain3/1 -> Sum/1
  [poc_in] -> Sum1/1
  Sum1/1 -> [LIL]
  PID Controller/1 -> Display5/1, Saturation/1, Display7/1
  Gain4/1 -> Display6/1, PID Controller/1
  Dead Zone Dynamic/1 -> Display4/1, Gain4/1
  E_PID: 0 - 100%/1 -> Display1/1, Sum/2
  ref_P:0 - 187/1 -> Display/1, Gain3/1
  [LIH] -> Dead Zone Dynamic/1
  Saturation/1 -> POC_out/1
  Sum/1 -> Display2/1, [poc_in]
  Gain2/1 -> Dead Zone Dynamic/2
  Constant/1 -> Sum2/2, Sum1/2
  [poc_in] -> Sum2/1
  P: 0 - 187/1 -> Display3/1, Gain2/1

== system CDA/U2/Regulador1/PID ==
  f : Inport
  Dead Zone : DeadZone  LowerValue=100-0.01  UpperValue=100+0.01  SaturateOnIntegerOverflow=on
  Derivative : Derivative
  Gain : Gain  Gain=1/tx
  Gain1 : Gain  Gain=kp
  Gain2 : Gain  Gain=td
  Gain3 : Gain  Gain=bp
  Gain4 : Gain  Gain=-1
  Gain5 : Gain  Gain=100
  IC1 : InitialCondition  Value=100
  Integrator : Integrator
  Saturation : Saturate  UpperLimit=2.5  LowerLimit=-2.5
  Sum1 : Sum  Inputs=++|
  Sum2 : Sum  Inputs=++|
  Sum3 : Sum  Inputs=|+-
  Transfer Fcn1 : TransferFcn  Denominator=[t3 1]
  e_pid : Outport
  wires:
  Saturation/1 -> e_pid/1
  Transfer Fcn1/1 -> Integrator/1, Gain2/1
  Gain2/1 -> Sum2/1
  Sum1/1 -> Transfer Fcn1/1
  Dead Zone/1 -> Gain4/1
  Integrator/1 -> Sum2/2, Gain3/1
  Gain3/1 -> Sum3/2
  f/1 -> Gain5/1
  Derivative/1 -> Gain1/1
  IC1/1 -> Dead Zone/1
  Gain4/1 -> Sum3/1, Derivative/1
  Gain/1 -> Sum1/2
  Gain1/1 -> Sum1/1
  Sum2/1 -> Saturation/1
  Sum3/1 -> Gain/1
  Gain5/1 -> IC1/1

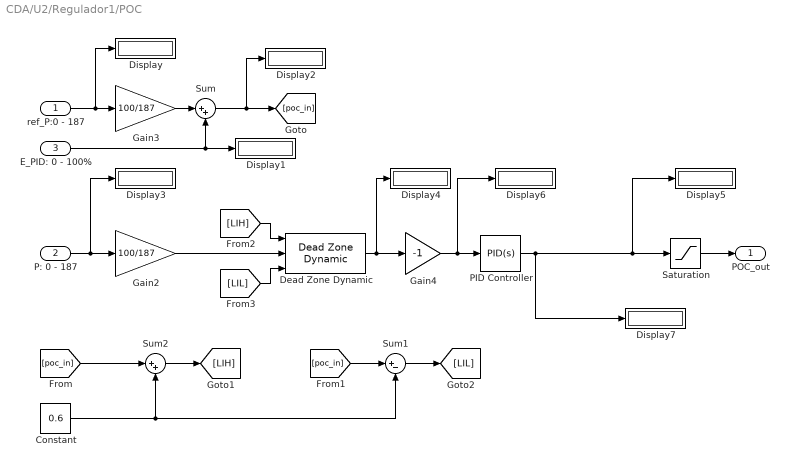
== system CDA/U2/Regulador1/POC ==
  ref_P:0 - 187 : Inport
  P: 0 - 187 : Inport  Port=2
  E_PID: 0 - 100% : Inport  Port=3
  Constant : Constant  Value=0.6
  Dead Zone Dynamic : simulink/Discontinuities/Dead Zone Dynamic
      settings: SourceProductBaseCode=SL
  Display{,1..7} (8 alike) : Display
  Gain2 : Gain  Gain=100/187
  Gain3 : Gain  Gain=100/187
  Gain4 : Gain  Gain=-1
  PID Controller : simulink/Continuous/PID Controller  Controller=PID  Form=Parallel  TimeDomain=Continuous-time  UseExternalTs=off  SampleTime=-1  IntegratorMethod=Forward Euler  FilterMethod=Forward Euler  ControllerParametersSource=internal  P=kp_poc  I=kp_poc/tn_poc  D=0  UseFilter=on  N=100  TunerSelectOption=Transfer Function Based (PID Tuner App)  InitialConditionSource=internal  InitialConditionForIntegrator=poc_i_u2  InitialConditionForFilter=0  DifferentiatorICPrevScaledInput=0  ExternalReset=none  TrackingMode=off  Kt=1  LimitOutput=off  UpperSaturationLimit=inf  LowerSaturationLimit=-inf  LinearizeAsGain=on  AntiWindupMode=none  Kb=1  POutMin=[]  POutMax=[]  IOutMin=[]  IOutMax=[]  DOutMin=[]  DOutMax=[]  NOutMin=[]  NOutMax=[]  SumOutMin=[]  SumOutMax=[]  SaturationOutMin=[]  SaturationOutMax=[]  PParamMin=[]  PParamMax=[]  IParamMin=[]  IParamMax=[]  DParamMin=[]  DParamMax=[]  NParamMin=[]  NParamMax=[]  KbParamMin=[]  KbParamMax=[]  KtParamMin=[]  KtParamMax=[]  KbOutMin=[]  KbOutMax=[]  KtOutMin=[]  KtOutMax=[]  IntegratorOutMin=[]  IntegratorOutMax=[]  FilterOutMin=[]  FilterOutMax=[]  SumI1OutMin=[]  SumI1OutMax=[]  SumI2OutMin=[]  SumI2OutMax=[]  SumI3OutMin=[]  SumI3OutMax=[]  SumI4OutMin=[]  SumI4OutMax=[]  SumDOutMin=[]  SumDOutMax=[]  DifferentiatorOutMin=[]  DifferentiatorOutMax=[]  FilterDiffOutCoefMin=[]  FilterDiffOutCoefMax=[]  ReciprocalOutMin=[]  ReciprocalOutMax=[]  SumDenOutMin=[]  SumDenOutMax=[]  SumNumOutMin=[]  SumNumOutMax=[]  DivideOutMin=[]  DivideOutMax=[]  UdiffTsProdOutMin=[]  UdiffTsProdOutMax=[]  NTsProdOutMin=[]  NTsProdOutMax=[]  UintegralTsProdOutMin=[]  UintegralTsProdOutMax=[]  UngainTsProdOutMin=[]  UngainTsProdOutMax=[]  IntegratorContinuousStateAttributes=''  IntegratorStateMustResolveToSignalObject=off  IntegratorRTWStateStorageClass=Auto  FilterContinuousStateAttributes=''  FilterStateMustResolveToSignalObject=off  FilterRTWStateStorageClass=Auto  ParallelPVariant=InternalParameters  IdealPVariant=Disabled  IVariant=InternalParameters  DVariant=InternalParameters  IntegratorVariant=Continuous  SatVariant=Disabled  AWVariant=Passthrough  PCopyVariant=Disabled  TRVariant=Disabled  FdbkBlocksVariant=Forward  IdealPFdbkVariant=Disabled  SatFdbkVariant=Disabled  DerivativeFilterVariant=ContFilter  NVariant=InternalParameters  NCopyVariant=Disabled  FilterICVariant=InternalICsFilter  IntegratorICVariant=InternalICs  ExternalResetVariant=Disabled  TRSumVariant=Passthrough  SumFdbkVariant=Disabled  SumVariant=Sum_PID  TsampFilterVariant=InternalTs  TsampNgainVariant=Passthrough  TsampIntegralVariant=Passthrough
  Saturation : Saturate  UpperLimit=120  LowerLimit=-120  ZeroCross=off
  Sum : Sum  Inputs=|++
  Sum1 : Sum  Inputs=|+-
  Sum2 : Sum  Inputs=|++
  POC_out : Outport
  wires:
  Sum2/1 -> [LIH]
  [LIL] -> Dead Zone Dynamic/3
  Gain3/1 -> Sum/1
  [poc_in] -> Sum1/1
  Sum1/1 -> [LIL]
  PID Controller/1 -> Display5/1, Saturation/1, Display7/1
  Gain4/1 -> Display6/1, PID Controller/1
  Dead Zone Dynamic/1 -> Display4/1, Gain4/1
  E_PID: 0 - 100%/1 -> Display1/1, Sum/2
  ref_P:0 - 187/1 -> Display/1, Gain3/1
  [LIH] -> Dead Zone Dynamic/1
  Saturation/1 -> POC_out/1
  Sum/1 -> Display2/1, [poc_in]
  Gain2/1 -> Dead Zone Dynamic/2
  Constant/1 -> Sum2/2, Sum1/2
  [poc_in] -> Sum2/1
  P: 0 - 187/1 -> Display3/1, Gain2/1

== system CDA/U3/Regulador1/PID ==
  f : Inport
  Dead Zone : DeadZone  LowerValue=100-0.01  UpperValue=100+0.01  SaturateOnIntegerOverflow=on
  Derivative : Derivative
  Gain : Gain  Gain=1/tx
  Gain1 : Gain  Gain=kp
  Gain2 : Gain  Gain=td
  Gain3 : Gain  Gain=bp
  Gain4 : Gain  Gain=-1
  Gain5 : Gain  Gain=100
  IC1 : InitialCondition  Value=100
  Integrator : Integrator
  Saturation : Saturate  UpperLimit=2.5  LowerLimit=-2.5
  Sum1 : Sum  Inputs=++|
  Sum2 : Sum  Inputs=++|
  Sum3 : Sum  Inputs=|+-
  Transfer Fcn1 : TransferFcn  Denominator=[t3 1]
  e_pid : Outport
  wires:
  Saturation/1 -> e_pid/1
  Transfer Fcn1/1 -> Integrator/1, Gain2/1
  Gain2/1 -> Sum2/1
  Sum1/1 -> Transfer Fcn1/1
  Dead Zone/1 -> Gain4/1
  Integrator/1 -> Sum2/2, Gain3/1
  Gain3/1 -> Sum3/2
  f/1 -> Gain5/1
  Derivative/1 -> Gain1/1
  IC1/1 -> Dead Zone/1
  Gain4/1 -> Sum3/1, Derivative/1
  Gain/1 -> Sum1/2
  Gain1/1 -> Sum1/1
  Sum2/1 -> Saturation/1
  Sum3/1 -> Gain/1
  Gain5/1 -> IC1/1

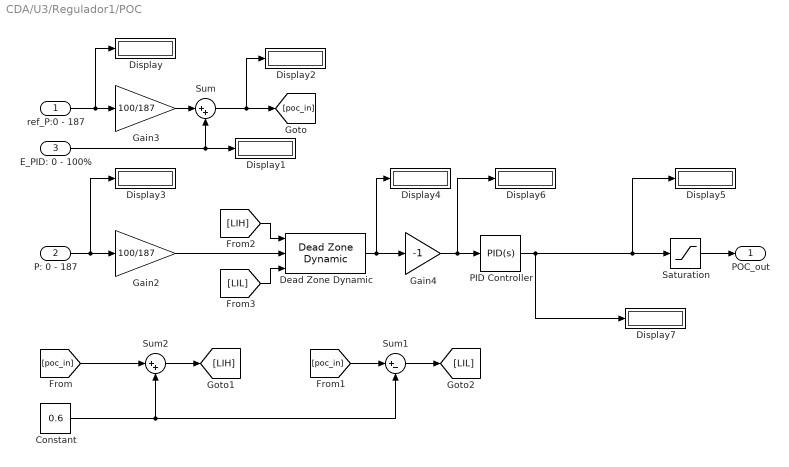
== system CDA/U3/Regulador1/POC ==
  ref_P:0 - 187 : Inport
  P: 0 - 187 : Inport  Port=2
  E_PID: 0 - 100% : Inport  Port=3
  Constant : Constant  Value=0.6
  Dead Zone Dynamic : simulink/Discontinuities/Dead Zone Dynamic
      settings: SourceProductBaseCode=SL
  Display{,1..7} (8 alike) : Display
  Gain2 : Gain  Gain=100/187
  Gain3 : Gain  Gain=100/187
  Gain4 : Gain  Gain=-1
  PID Controller : simulink/Continuous/PID Controller  Controller=PID  Form=Parallel  TimeDomain=Continuous-time  UseExternalTs=off  SampleTime=-1  IntegratorMethod=Forward Euler  FilterMethod=Forward Euler  ControllerParametersSource=internal  P=kp_poc  I=kp_poc/tn_poc  D=0  UseFilter=on  N=100  TunerSelectOption=Transfer Function Based (PID Tuner App)  InitialConditionSource=internal  InitialConditionForIntegrator=poc_i_u3  InitialConditionForFilter=0  DifferentiatorICPrevScaledInput=0  ExternalReset=none  TrackingMode=off  Kt=1  LimitOutput=off  UpperSaturationLimit=inf  LowerSaturationLimit=-inf  LinearizeAsGain=on  AntiWindupMode=none  Kb=1  POutMin=[]  POutMax=[]  IOutMin=[]  IOutMax=[]  DOutMin=[]  DOutMax=[]  NOutMin=[]  NOutMax=[]  SumOutMin=[]  SumOutMax=[]  SaturationOutMin=[]  SaturationOutMax=[]  PParamMin=[]  PParamMax=[]  IParamMin=[]  IParamMax=[]  DParamMin=[]  DParamMax=[]  NParamMin=[]  NParamMax=[]  KbParamMin=[]  KbParamMax=[]  KtParamMin=[]  KtParamMax=[]  KbOutMin=[]  KbOutMax=[]  KtOutMin=[]  KtOutMax=[]  IntegratorOutMin=[]  IntegratorOutMax=[]  FilterOutMin=[]  FilterOutMax=[]  SumI1OutMin=[]  SumI1OutMax=[]  SumI2OutMin=[]  SumI2OutMax=[]  SumI3OutMin=[]  SumI3OutMax=[]  SumI4OutMin=[]  SumI4OutMax=[]  SumDOutMin=[]  SumDOutMax=[]  DifferentiatorOutMin=[]  DifferentiatorOutMax=[]  FilterDiffOutCoefMin=[]  FilterDiffOutCoefMax=[]  ReciprocalOutMin=[]  ReciprocalOutMax=[]  SumDenOutMin=[]  SumDenOutMax=[]  SumNumOutMin=[]  SumNumOutMax=[]  DivideOutMin=[]  DivideOutMax=[]  UdiffTsProdOutMin=[]  UdiffTsProdOutMax=[]  NTsProdOutMin=[]  NTsProdOutMax=[]  UintegralTsProdOutMin=[]  UintegralTsProdOutMax=[]  UngainTsProdOutMin=[]  UngainTsProdOutMax=[]  IntegratorContinuousStateAttributes=''  IntegratorStateMustResolveToSignalObject=off  IntegratorRTWStateStorageClass=Auto  FilterContinuousStateAttributes=''  FilterStateMustResolveToSignalObject=off  FilterRTWStateStorageClass=Auto  ParallelPVariant=InternalParameters  IdealPVariant=Disabled  IVariant=InternalParameters  DVariant=InternalParameters  IntegratorVariant=Continuous  SatVariant=Disabled  AWVariant=Passthrough  PCopyVariant=Disabled  TRVariant=Disabled  FdbkBlocksVariant=Forward  IdealPFdbkVariant=Disabled  SatFdbkVariant=Disabled  DerivativeFilterVariant=ContFilter  NVariant=InternalParameters  NCopyVariant=Disabled  FilterICVariant=InternalICsFilter  IntegratorICVariant=InternalICs  ExternalResetVariant=Disabled  TRSumVariant=Passthrough  SumFdbkVariant=Disabled  SumVariant=Sum_PID  TsampFilterVariant=InternalTs  TsampNgainVariant=Passthrough  TsampIntegralVariant=Passthrough
  Saturation : Saturate  UpperLimit=120  LowerLimit=-120  ZeroCross=off
  Sum : Sum  Inputs=|++
  Sum1 : Sum  Inputs=|+-
  Sum2 : Sum  Inputs=|++
  POC_out : Outport
  wires:
  Sum2/1 -> [LIH]
  [LIL] -> Dead Zone Dynamic/3
  Gain3/1 -> Sum/1
  [poc_in] -> Sum1/1
  Sum1/1 -> [LIL]
  PID Controller/1 -> Display5/1, Saturation/1, Display7/1
  Gain4/1 -> Display6/1, PID Controller/1
  Dead Zone Dynamic/1 -> Display4/1, Gain4/1
  E_PID: 0 - 100%/1 -> Display1/1, Sum/2
  ref_P:0 - 187/1 -> Display/1, Gain3/1
  [LIH] -> Dead Zone Dynamic/1
  Saturation/1 -> POC_out/1
  Sum/1 -> Display2/1, [poc_in]
  Gain2/1 -> Dead Zone Dynamic/2
  Constant/1 -> Sum2/2, Sum1/2
  [poc_in] -> Sum2/1
  P: 0 - 187/1 -> Display3/1, Gain2/1
